simulink model "SimulationModel"  (R2015a)
settings: Solver=ode3  SolverMode=SingleTasking  StartTime=0.0  StopTime=180  FixedStep=Ts  RelTol=1e-3
PostLoadFcn:
  | loadRobotParameters
StartFcn:
  | reset(SimDisplay.getInstance());
undefined symbols (not defined in the file): AxleLength, do_one_run, EncL_init, EncR_init, EncRes, lcam, motorL, motorR, motorX, pcam, SitesPositions, slip_intensity, startPos, TauMotor, theta0, Ts, WheelRadius
libraries: pil_lib x2, simulink x1, realtime_pacer_lib x1, cstblocks x1
CloseFcn:
  | delete(SimDisplay.getInstance());
settings Model: PauseTimes=14  CovSFcnEnable=off  ExtModeTrigDuration=2  Creator=gpacitti  LastModifiedBy=Ye
settings DataIOCC: SaveOutput=off  DSMLogging=off  SaveTime=off
settings OptimizationCC: ExpressionDepthLimit=2147483647  OptimizeModelRefInitCode=on  LifeSpan=1  MaxStackSize=64
settings DebuggingCC: UnderspecifiedInitializationDetection=Classic  MergeDetectMultiDrivingBlocksExec=none  MultiTaskDSMMsg=warning  MultiTaskCondExecSysMsg=none  ParameterPrecisionLossMsg=none  StateNameClashWarn=warning
settings HardwareCC: ProdLargestAtomicInteger=Long  ProdLargestAtomicFloat=Double  ProdEndianess=LittleEndian  ProdHWDeviceType=ARM Compatible->ARM Cortex
settings RTWCC: SystemTargetFile=ert.tlc  TLCOptions=-aInlineSetEventsForThisBaseRateFcn=TLC_FALSE -aSuppressMultiTaskScheduler=TLC_FALSE  TemplateMakefile=ert_default_tmf  Description=Embedded Coder  RTWVerbose=off  Toolchain=GNU Tools for ARM Embedded Processors  CreateSILPILBlock=PIL  CodeExecutionProfiling=on  CodeProfilingSaveOptions=AllData
settings CodeAppCC: IgnoreCustomStorageClasses=off  CustomSymbolStrType=$N$R$M  InternalIdentifier=Classic
settings ERTTargetCC: CodeReplacementLibrary=ARM Cortex-M  GenerateSampleERTMain=off  ParMdlRefBuildCompliant=on  CompOptLevelCompliant=on  ConcurrentExecutionCompliant=on  ERTFirstTimeCompliant=on  SupportContinuousTime=off  ModelStepFunctionPrototypeControlCompliant=on  CPPClassGenCompliant=on  InlinedParameterPlacement=Hierarchical
settings ConfigComp: Description=Design Verifier Custom Configuration Component  DVMaxTestCaseSteps=500  DVTestSuiteOptimization=CombinedObjectives (Nonlinear Extended)  DVDetectActiveLogic=on

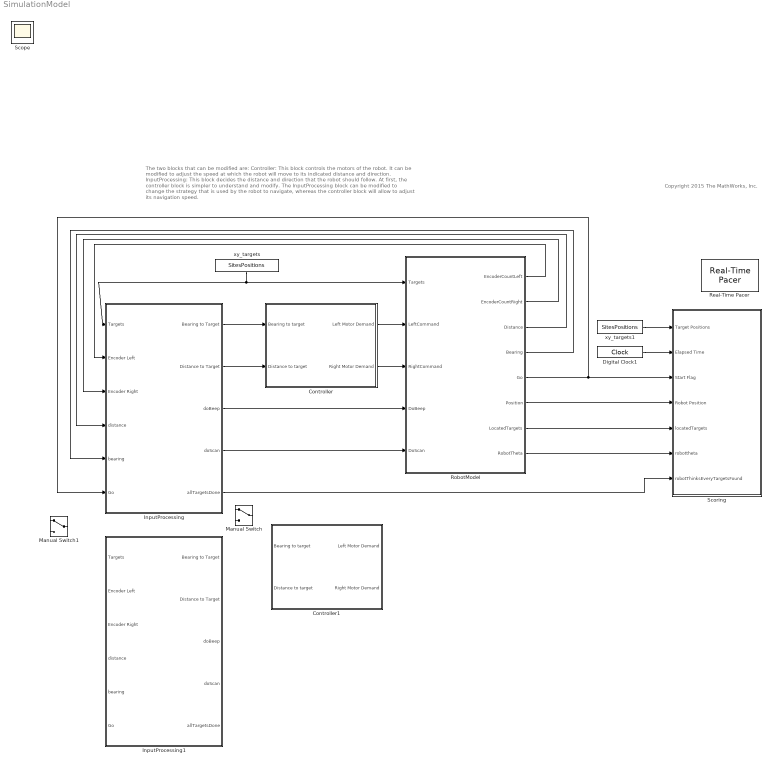
== system SimulationModel ==
  note: Copyright 2015 The MathWorks, Inc.
  note: The two blocks that can be modified are:
      | Controller: This block controls the motors of the robot. It can be modified to adjust the speed at which the robot will move to its indicated distance and direction.
      | InputProcessing: This block decides the distance and direction that the robot should follow.
      |
      | At first, the controller block is simpler to understand and modify.
      | The InputProcessing block can be modified to change the strategy that is used by the robot to navigate, whereas the controller block will allow to adjust its navigation speed.
  Controller : Subsystem  TreatAsAtomicUnit=on
      mask Display: image('Arduino_Mega_2560.jpg',[0.75/2,0.3,0.25,0.4]);
  Controller1 : Subsystem  DialogController=pil_create_dialog  LoadFcn=|
      | try
      |    if ~strcmp(rtw.pil.getPILVersion, '6.8 (R2015a)_12')
      |       set_param(gcb, 'DialogController', '');
      |       set_param(gcb, 'DialogControllerArgs', '');
      |    end
      | catch e
      |       set_param(gcb, 'DialogController', '');
      |       set_param(gcb, 'DialogControllerArgs', '');
      | end
      mask help: PIL:pil:XILBlockMaskDesc
      mask Display: disp('PIL');
  Digital Clock1 : DigitalClock  SampleTime=Ts
  InputProcessing : Subsystem
      mask Display: image('Arduino_Mega_2560.jpg',[0.75/2,0.3,0.25,0.3]);
  InputProcessing1 : Subsystem  DialogController=pil_create_dialog  LoadFcn=|
      | try
      |    if ~strcmp(rtw.pil.getPILVersion, '6.8 (R2015a)_12')
      |       set_param(gcb, 'DialogController', '');
      |       set_param(gcb, 'DialogControllerArgs', '');
      |    end
      | catch e
      |       set_param(gcb, 'DialogController', '');
      |       set_param(gcb, 'DialogControllerArgs', '');
      | end
      mask help: PIL:pil:XILBlockMaskDesc
      mask Display: disp('PIL');
  Manual Switch : ManualSwitch
  Manual Switch1 : ManualSwitch
  Real-Time Pacer : realtime_pacer_lib/Real-Time Pacer  simTimePerRealTime=1
  RobotModel : Subsystem
      mask Display: image('robot_3d.jpg',[0.25,0.35,0.45,0.25]);
  Scoring : Subsystem
      mask Display: image('juge.jpg',[0.45,0.3,0.5,0.25]);
  xy_targets : Constant  Value=SitesPositions  OutDataTypeStr=single
  xy_targets1 : Constant  Value=SitesPositions  OutDataTypeStr=single
  Scope : Scope
      settings: MaxDataPoints=7500
  wires:
  RobotModel/2(EncoderCountRight) -> InputProcessing/3(Encoder Right)
  RobotModel/1(EncoderCountLeft) -> InputProcessing/2(Encoder Left)
  xy_targets/1 -> InputProcessing/1(Targets), RobotModel/1(Targets)
  RobotModel/6(Position) -> Scoring/4(Robot Position)
  InputProcessing/2(Distance to Target) -> Controller/2(Distance to target)
  InputProcessing/1(Bearing to Target) -> Controller/1(Bearing to target)
  Controller/1(Left Motor Demand) -> RobotModel/2(LeftCommand)
  Controller/2(Right Motor Demand) -> RobotModel/3(RightCommand)
  RobotModel/5(Go) -> InputProcessing/6(Go), Scoring/3(Start Flag)
  Digital Clock1/1 -> Scoring/2(Elapsed Time)
  RobotModel/3(Distance) -> InputProcessing/4(distance)
  RobotModel/4(Bearing) -> InputProcessing/5(bearing)
  RobotModel/7(LocatedTargets) -> Scoring/5(locatedTargets)
  RobotModel/8(RobotTheta) -> Scoring/6(robottheta)
  InputProcessing/5(allTargetsDone) -> Scoring/7(robotThinksEveryTargetsFound)
  xy_targets1/1 -> Scoring/1(Target Positions)
  InputProcessing/3(doBeep) -> RobotModel/4(DoBeep)
  InputProcessing/4(doScan) -> RobotModel/5(DoScan)

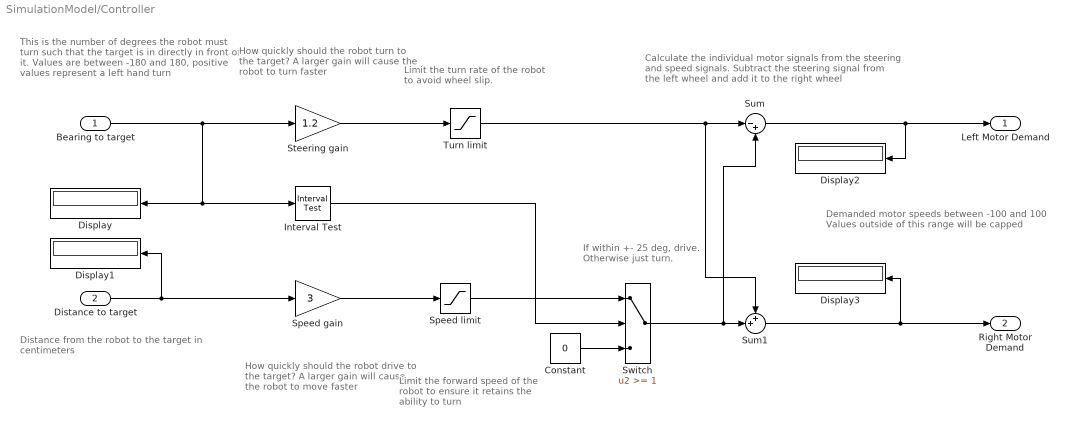
== system SimulationModel/Controller ==
  note: This is the number of degrees the robot
      | must turn such that the target is in directly
      | in front of it.
      | Values are between -180 and 180,
      | positive values represent a left hand turn
  note: Distance from the robot to the target
      | in centimeters
  note: Demanded motor speeds between -100 and 100
      | Values outside of this range will be capped
  note: How quickly should the robot turn
      | to the target? A larger gain will
      |  cause the robot to turn faster
  note: How quickly should the robot
      | drive to the target? A larger gain
      | will cause the robot to move
      | faster
  note: Limit the forward speed of the
      | robot to ensure it retains the
      | ability to turn
  note: Calculate the individual motor signals from the
      | steering and speed signals. Subtract the steering
      | signal from the left wheel and add it to the right
      | wheel
  note: If within +- 25 deg, drive.
      | Otherwise just turn.
  note: Limit the turn rate of the
      | robot to avoid wheel slip.
  Bearing to target : Inport  OutDataTypeStr=single
  Distance to target : Inport  Port=2  PortDimensions=1  SampleTime=Ts
  Constant : Constant  Value=0  OutDataTypeStr=single
  Display{,1..3} (4 alike) : Display
  Interval Test : simulink/Logic and Bit Operations/Interval Test  IntervalClosedRight=on  uplimit=25  IntervalClosedLeft=on  lowlimit=-25  OutDataTypeStr=boolean
      settings: AttributesFormatString=|
      | Upper = %<uplimit>
      | Lower = %<lowlimit>
  Speed gain : Gain  Gain=3
  Speed limit : Saturate  UpperLimit=40  LowerLimit=0
      settings: AttributesFormatString=|
      | Upper = %<UpperLimit>
      | Lower = %<LowerLimit>
  Steering gain : Gain  Gain=1.2
  Sum : Sum  Inputs=|-+
  Sum1 : Sum  Inputs=++|
  Switch : Switch  Threshold=1
  Turn limit : Saturate  UpperLimit=50  LowerLimit=-50
      settings: AttributesFormatString=|
      | Upper = %<UpperLimit>
      | Lower = %<LowerLimit>
  Left Motor Demand : Outport  OutDataTypeStr=single
  Right Motor Demand : Outport  Port=2  OutDataTypeStr=single
  wires:
  Speed limit/1 -> Switch/1
  Turn limit/1 -> Sum1/1, Sum/1
  Constant/1 -> Switch/3
  Interval Test/1 -> Switch/2
  Switch/1 -> Sum1/2, Sum/2
  Sum/1 -> Display2/1, Left Motor Demand/1
  Sum1/1 -> Display3/1, Right Motor Demand/1
  Steering gain/1 -> Turn limit/1
  Distance to target/1 -> Speed gain/1, Display1/1
  Speed gain/1 -> Speed limit/1
  Bearing to target/1 -> Interval Test/1, Display/1, Steering gain/1

== system SimulationModel/Controller1 ==
  Bearing to target : Inport  OutDataTypeStr=single
  Distance to target : Inport  Port=2  PortDimensions=1  SampleTime=Ts
  Controller_sfcn : pil_lib/PIL Block  SimulationMode=PIL  IsTopModelPIL=off  CodeDir=D:\Dropbox\Phd\AutomaticScriptForSubRegions\MarsRover2014\work\Controller_ert_rtw  ConfigName=ARM Cortex-M3 (QEMU)
  __InputSSForSFun__ : Subsystem
  __OutputSSForSFun__ : Subsystem
  Left Motor Demand : Outport  OutDataTypeStr=single
  Right Motor Demand : Outport  Port=2  OutDataTypeStr=single
  wires:
  __OutputSSForSFun__/2(Right Motor Demand) -> Right Motor Demand/1
  __OutputSSForSFun__/1(Left Motor Demand) -> Left Motor Demand/1
  Controller_sfcn/2 -> __OutputSSForSFun__/2(__UniqueInportName__2__)
  Controller_sfcn/1 -> __OutputSSForSFun__/1(__UniqueInportName__1__)
  __InputSSForSFun__/2(__UniqueOutportName__2__) -> Controller_sfcn/2
  __InputSSForSFun__/1(__UniqueOutportName__1__) -> Controller_sfcn/1
  Distance to target/1 -> __InputSSForSFun__/2(Distance to target)
  Bearing to target/1 -> __InputSSForSFun__/1(Bearing to target)

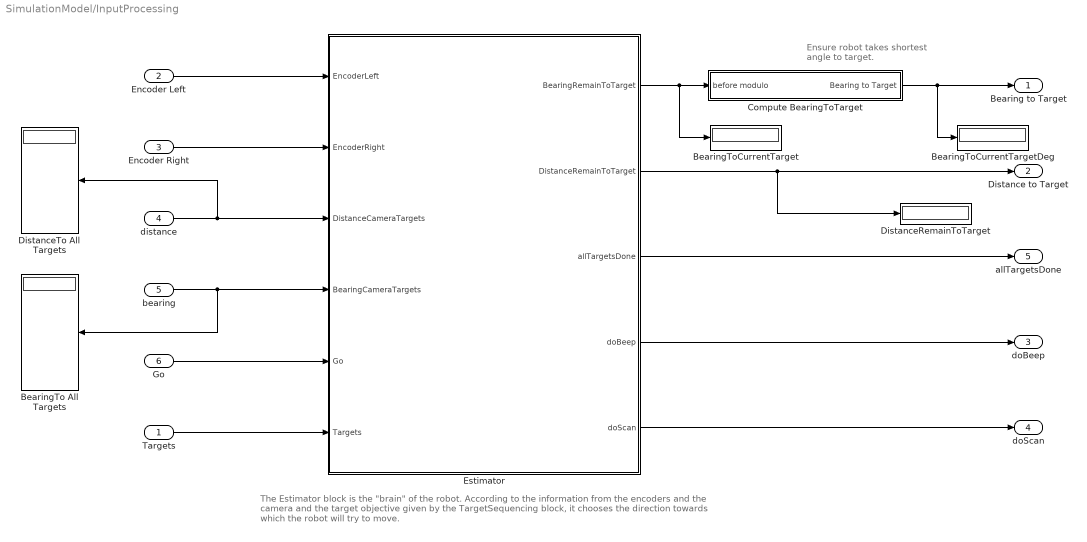
== system SimulationModel/InputProcessing ==
  note: The Estimator block is the "brain" of the robot. According to the information from the encoders and the camera and the
      | target objective given by the TargetSequencing block, it chooses the direction towards which the robot will try to move.
  note: Ensure robot takes shortest
      | angle to target.
  Targets : Inport
  Encoder Left : Inport  Port=2  OutDataTypeStr=int32
  Encoder Right : Inport  Port=3  OutDataTypeStr=int32
  distance : Inport  Port=4
  bearing : Inport  Port=5
  Go : Inport  Port=6
  BearingTo All Targets : Display
  BearingToCurrentTarget : Display
  BearingToCurrentTargetDeg : Display
  Compute BearingToTarget : Subsystem
  DistanceRemainToTarget : Display
  DistanceTo All Targets : Display
  Estimator : Stateflow chart  TreatAsAtomicUnit=on
  Bearing to Target : Outport  SampleTime=Ts
  Distance to Target : Outport  Port=2
  doBeep : Outport  Port=3
  doScan : Outport  Port=4
  allTargetsDone : Outport  Port=5
  wires:
  distance/1 -> DistanceTo All Targets/1, Estimator/3(DistanceCameraTargets)
  bearing/1 -> BearingTo All Targets/1, Estimator/4(BearingCameraTargets)
  Compute BearingToTarget/1(Bearing to Target) -> BearingToCurrentTargetDeg/1, Bearing to Target/1
  Estimator/2(DistanceRemainToTarget) -> DistanceRemainToTarget/1, Distance to Target/1
  Estimator/1(BearingRemainToTarget) -> Compute BearingToTarget/1(before modulo), BearingToCurrentTarget/1
  Encoder Right/1 -> Estimator/2(EncoderRight)
  Encoder Left/1 -> Estimator/1(EncoderLeft)
  Targets/1 -> Estimator/6(Targets)
  Go/1 -> Estimator/5(Go)
  Estimator/3(allTargetsDone) -> allTargetsDone/1
  Estimator/4(doBeep) -> doBeep/1
  Estimator/5(doScan) -> doScan/1

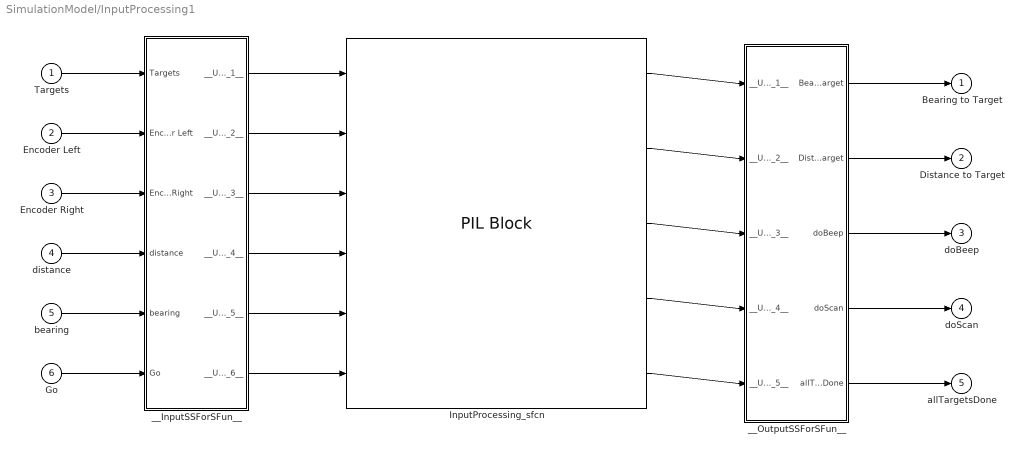
== system SimulationModel/InputProcessing1 ==
  Targets : Inport
  Encoder Left : Inport  Port=2  OutDataTypeStr=int32
  Encoder Right : Inport  Port=3  OutDataTypeStr=int32
  distance : Inport  Port=4
  bearing : Inport  Port=5
  Go : Inport  Port=6
  InputProcessing_sfcn : pil_lib/PIL Block  SimulationMode=PIL  IsTopModelPIL=off  CodeDir=D:\Dropbox\Phd\AutomaticScriptForSubRegions\MarsRover2014\work\InputProcessing_ert_rtw  ConfigName=ARM Cortex-M3 (QEMU)
  __InputSSForSFun__ : Subsystem
  __OutputSSForSFun__ : Subsystem
  Bearing to Target : Outport  SampleTime=Ts
  Distance to Target : Outport  Port=2
  doBeep : Outport  Port=3
  doScan : Outport  Port=4
  allTargetsDone : Outport  Port=5
  wires:
  __OutputSSForSFun__/5(allTargetsDone) -> allTargetsDone/1
  __OutputSSForSFun__/4(doScan) -> doScan/1
  __OutputSSForSFun__/3(doBeep) -> doBeep/1
  __OutputSSForSFun__/2(Distance to Target) -> Distance to Target/1
  __OutputSSForSFun__/1(Bearing to Target) -> Bearing to Target/1
  InputProcessing_sfcn/5 -> __OutputSSForSFun__/5(__UniqueInportName__5__)
  InputProcessing_sfcn/4 -> __OutputSSForSFun__/4(__UniqueInportName__4__)
  InputProcessing_sfcn/3 -> __OutputSSForSFun__/3(__UniqueInportName__3__)
  InputProcessing_sfcn/2 -> __OutputSSForSFun__/2(__UniqueInportName__2__)
  InputProcessing_sfcn/1 -> __OutputSSForSFun__/1(__UniqueInportName__1__)
  __InputSSForSFun__/6(__UniqueOutportName__6__) -> InputProcessing_sfcn/6
  __InputSSForSFun__/5(__UniqueOutportName__5__) -> InputProcessing_sfcn/5
  __InputSSForSFun__/4(__UniqueOutportName__4__) -> InputProcessing_sfcn/4
  __InputSSForSFun__/3(__UniqueOutportName__3__) -> InputProcessing_sfcn/3
  __InputSSForSFun__/2(__UniqueOutportName__2__) -> InputProcessing_sfcn/2
  __InputSSForSFun__/1(__UniqueOutportName__1__) -> InputProcessing_sfcn/1
  Go/1 -> __InputSSForSFun__/6(Go)
  bearing/1 -> __InputSSForSFun__/5(bearing)
  distance/1 -> __InputSSForSFun__/4(distance)
  Encoder Right/1 -> __InputSSForSFun__/3(Encoder Right)
  Encoder Left/1 -> __InputSSForSFun__/2(Encoder Left)
  Targets/1 -> __InputSSForSFun__/1(Targets)

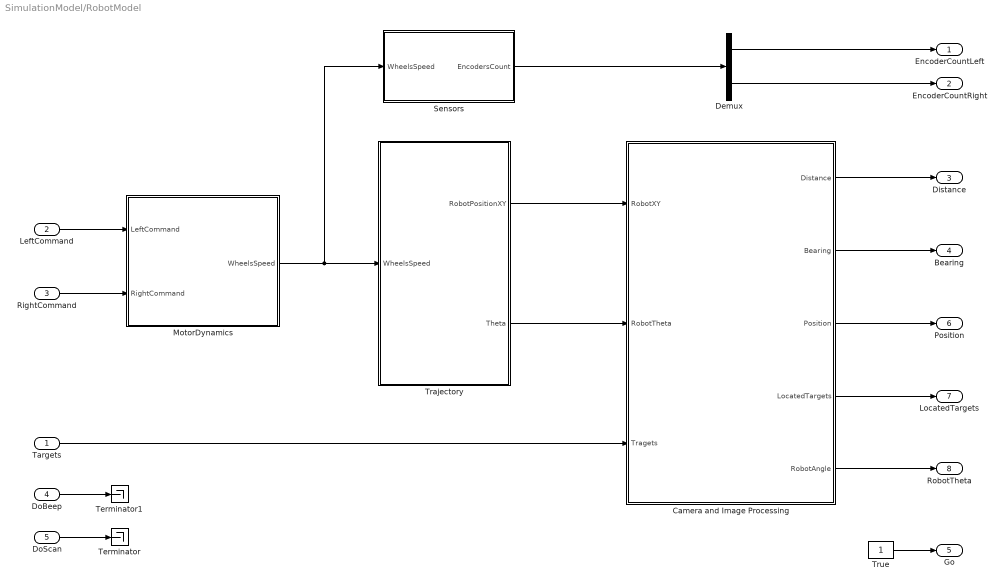
== system SimulationModel/RobotModel ==
  Targets : Inport
  LeftCommand : Inport  Port=2  SampleTime=0
  RightCommand : Inport  Port=3  SampleTime=0
  DoBeep : Inport  Port=4  SampleTime=0
  DoScan : Inport  Port=5  SampleTime=0
  Camera and Image Processing : Subsystem
  Demux : Demux  Outputs=2
  MotorDynamics : Subsystem
  Sensors : Subsystem
  Terminator : Terminator
  Terminator1 : Terminator
  Trajectory : Subsystem
  True : Constant  OutMin=0  OutMax=1  OutDataTypeStr=boolean  SampleTime=0.1
  EncoderCountLeft : Outport  OutDataTypeStr=int32
  EncoderCountRight : Outport  Port=2  OutDataTypeStr=int32
  Distance : Outport  Port=3  OutDataTypeStr=int16
  Bearing : Outport  Port=4  OutDataTypeStr=int8
  Go : Outport  Port=5
  Position : Outport  Port=6
  LocatedTargets : Outport  Port=7
  RobotTheta : Outport  Port=8
  wires:
  Trajectory/2(Theta) -> Camera and Image Processing/2(RobotTheta)
  True/1 -> Go/1
  DoScan/1 -> Terminator/1
  DoBeep/1 -> Terminator1/1
  MotorDynamics/1(WheelsSpeed) -> Trajectory/1(WheelsSpeed), Sensors/1(WheelsSpeed)
  LeftCommand/1 -> MotorDynamics/1(LeftCommand)
  RightCommand/1 -> MotorDynamics/2(RightCommand)
  Sensors/1(EncodersCount) -> Demux/1
  Demux/1 -> EncoderCountLeft/1
  Demux/2 -> EncoderCountRight/1
  Targets/1 -> Camera and Image Processing/3(Tragets)
  Camera and Image Processing/1(Distance) -> Distance/1
  Camera and Image Processing/2(Bearing) -> Bearing/1
  Camera and Image Processing/3(Position) -> Position/1
  Camera and Image Processing/4(LocatedTargets) -> LocatedTargets/1
  Camera and Image Processing/5(RobotAngle) -> RobotTheta/1
  Trajectory/1(RobotPositionXY) -> Camera and Image Processing/1(RobotXY)

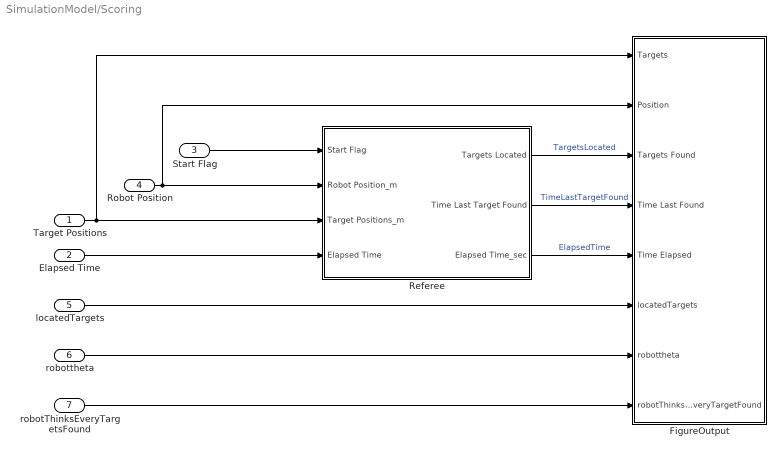
== system SimulationModel/Scoring ==
  Target Positions : Inport
  Elapsed Time : Inport  Port=2
  Start Flag : Inport  Port=3
  Robot Position : Inport  Port=4
  locatedTargets : Inport  Port=5
  robottheta : Inport  Port=6
  robotThinksEveryTargetsFound : Inport  Port=7
  FigureOutput : Subsystem  TreatAsAtomicUnit=on  SimViewingDevice=on
  Referee : Subsystem
      mask Display: % image(imread('referee.png'))
  wires:
  Referee/1(Targets Located) -> FigureOutput/3(Targets Found)  "TargetsLocated"
  Referee/2(Time Last Target Found) -> FigureOutput/4(Time Last Found)  "TimeLastTargetFound"
  Referee/3(Elapsed Time_sec) -> FigureOutput/5(Time Elapsed)  "ElapsedTime"
  Start Flag/1 -> Referee/1(Start Flag)
  Robot Position/1 -> Referee/2(Robot Position_m), FigureOutput/2(Position)
  Elapsed Time/1 -> Referee/4(Elapsed Time)
  Target Positions/1 -> FigureOutput/1(Targets), Referee/3(Target Positions_m)
  locatedTargets/1 -> FigureOutput/6(locatedTargets)
  robottheta/1 -> FigureOutput/7(robottheta)
  robotThinksEveryTargetsFound/1 -> FigureOutput/8(robotThinksEveryTargetFound)

== system SimulationModel/Controller1/__InputSSForSFun__ ==
  Bearing to target : Inport  OutDataTypeStr=single
  Distance to target : Inport  Port=2  PortDimensions=1  SampleTime=Ts
  __UniqueOutportName__1__ : Outport
  __UniqueOutportName__2__ : Outport  Port=2
  wires:
  Distance to target/1 -> __UniqueOutportName__2__/1
  Bearing to target/1 -> __UniqueOutportName__1__/1

== system SimulationModel/Controller1/__OutputSSForSFun__ ==
  __UniqueInportName__1__ : Inport
  __UniqueInportName__2__ : Inport  Port=2
  Left Motor Demand : Outport  OutDataTypeStr=single
  Right Motor Demand : Outport  Port=2  OutDataTypeStr=single
  wires:
  __UniqueInportName__2__/1 -> Right Motor Demand/1
  __UniqueInportName__1__/1 -> Left Motor Demand/1

== system SimulationModel/InputProcessing/Compute BearingToTarget ==
  before modulo : Inport
  Constant : Constant  Value=180  OutDataTypeStr=Inherit: Inherit via back propagation
  Constant1 : Constant  Value=360  OutDataTypeStr=Inherit: Inherit via back propagation
  Math Function1 : Math  Operator=mod  SaturateOnIntegerOverflow=on
  Sum10 : Sum  Inputs=-+|
  Sum7 : Sum  Inputs=++|
  Bearing to Target : Outport  SampleTime=Ts
  wires:
  before modulo/1 -> Sum7/2
  Sum10/1 -> Bearing to Target/1
  Math Function1/1 -> Sum10/2
  Constant1/1 -> Math Function1/2
  Sum7/1 -> Math Function1/1
  Constant/1 -> Sum10/1, Sum7/1

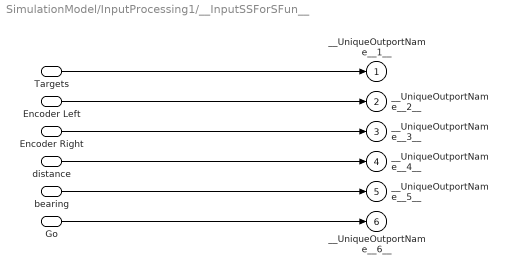
== system SimulationModel/InputProcessing1/__InputSSForSFun__ ==
  Targets : Inport
  Encoder Left : Inport  Port=2  OutDataTypeStr=int32
  Encoder Right : Inport  Port=3  OutDataTypeStr=int32
  distance : Inport  Port=4
  bearing : Inport  Port=5
  Go : Inport  Port=6
  __UniqueOutportName__1__ : Outport
  __UniqueOutportName__2__ : Outport  Port=2
  __UniqueOutportName__3__ : Outport  Port=3
  __UniqueOutportName__4__ : Outport  Port=4
  __UniqueOutportName__5__ : Outport  Port=5
  __UniqueOutportName__6__ : Outport  Port=6
  wires:
  Go/1 -> __UniqueOutportName__6__/1
  bearing/1 -> __UniqueOutportName__5__/1
  distance/1 -> __UniqueOutportName__4__/1
  Encoder Right/1 -> __UniqueOutportName__3__/1
  Encoder Left/1 -> __UniqueOutportName__2__/1
  Targets/1 -> __UniqueOutportName__1__/1

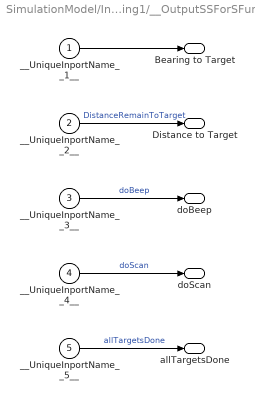
== system SimulationModel/InputProcessing1/__OutputSSForSFun__ ==
  __UniqueInportName__1__ : Inport
  __UniqueInportName__2__ : Inport  Port=2
  __UniqueInportName__3__ : Inport  Port=3
  __UniqueInportName__4__ : Inport  Port=4
  __UniqueInportName__5__ : Inport  Port=5
  Bearing to Target : Outport  SampleTime=Ts
  Distance to Target : Outport  Port=2
  doBeep : Outport  Port=3
  doScan : Outport  Port=4
  allTargetsDone : Outport  Port=5
  wires:
  __UniqueInportName__5__/1 -> allTargetsDone/1  "allTargetsDone"
  __UniqueInportName__4__/1 -> doScan/1  "doScan"
  __UniqueInportName__3__/1 -> doBeep/1  "doBeep"
  __UniqueInportName__2__/1 -> Distance to Target/1  "DistanceRemainToTarget"
  __UniqueInportName__1__/1 -> Bearing to Target/1

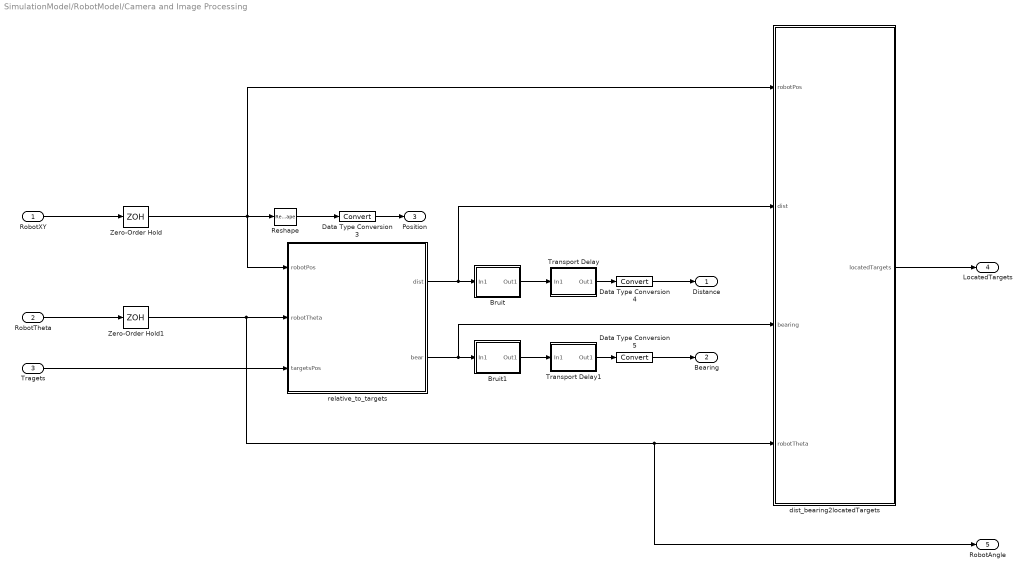
== system SimulationModel/RobotModel/Camera and Image Processing ==
  RobotXY : Inport
  RobotTheta : Inport  Port=2
  Tragets : Inport  Port=3
  Bruit : Subsystem
  Bruit1 : Subsystem
  Data Type Conversion3 : DataTypeConversion
  Data Type Conversion4 : DataTypeConversion
  Data Type Conversion5 : DataTypeConversion
  Reshape : Reshape  OutputDimensionality=Row vector (2-D)
  Transport Delay : Subsystem  mask{timeDelay=0.300, initialOutput=zeros(size(6,1),1), initialBufferSize=1024, useFixedBufferSize=off, directFeedthoughOfInputDuringLinearization=off, padeOrder=0}
      mask prompts: initialOutput "Initial output"; initialBufferSize "Initial buffer size"; useFixedBufferSize "Use fixed buffer size"; directFeedthoughOfInputDuringLinearization "Direct feedthough of input during linearization"; padeOrder "Pade order (for linearization):"
  Transport Delay1 : Subsystem  mask{timeDelay=0.300, initialOutput=zeros(size(6,1),1), initialBufferSize=1024, useFixedBufferSize=off, directFeedthoughOfInputDuringLinearization=off, padeOrder=0}
      mask prompts: initialOutput "Initial output"; initialBufferSize "Initial buffer size"; useFixedBufferSize "Use fixed buffer size"; directFeedthoughOfInputDuringLinearization "Direct feedthough of input during linearization"; padeOrder "Pade order (for linearization):"
  Zero-Order Hold : ZeroOrderHold  SampleTime=Ts
  Zero-Order Hold1 : ZeroOrderHold  SampleTime=Ts
  dist_bearing2locatedTargets : MATLAB Function  TreatAsAtomicUnit=on
  relative_to_targets : MATLAB Function  TreatAsAtomicUnit=on
  Distance : Outport  OutDataTypeStr=int16
  Bearing : Outport  Port=2  OutDataTypeStr=int8
  Position : Outport  Port=3
  LocatedTargets : Outport  Port=4
  RobotAngle : Outport  Port=5
  wires:
  RobotTheta/1 -> Zero-Order Hold1/1
  RobotXY/1 -> Zero-Order Hold/1
  Bruit/1(Out1) -> Transport Delay/1(In1)
  Transport Delay1/1(Out1) -> Data Type Conversion5/1
  Tragets/1 -> relative_to_targets/3(targetsPos)
  Data Type Conversion4/1 -> Distance/1
  Transport Delay/1(Out1) -> Data Type Conversion4/1
  Data Type Conversion5/1 -> Bearing/1
  Data Type Conversion3/1 -> Position/1
  Bruit1/1(Out1) -> Transport Delay1/1(In1)
  relative_to_targets/1(dist) -> dist_bearing2locatedTargets/2(dist), Bruit/1(In1)
  Reshape/1 -> Data Type Conversion3/1
  relative_to_targets/2(bear) -> dist_bearing2locatedTargets/3(bearing), Bruit1/1(In1)
  dist_bearing2locatedTargets/1(locatedTargets) -> LocatedTargets/1
  Zero-Order Hold/1 -> relative_to_targets/1(robotPos), dist_bearing2locatedTargets/1(robotPos), Reshape/1
  Zero-Order Hold1/1 -> RobotAngle/1, dist_bearing2locatedTargets/4(robotTheta), relative_to_targets/2(robotTheta)

== system SimulationModel/RobotModel/MotorDynamics ==
  LeftCommand : Inport
  RightCommand : Inport  Port=2
  Dynamics : cstblocks/LTI System  sys=tf(1,[TauMotor 1])*eye(2)  IC=[]
  Left_motor_table : Lookup_n-D  NumberOfTableDimensions=1  BreakpointsForDimension1=motorX  Table=motorL  ExtrapMethod=Clip  InternalRulePriority=Speed  OutDataTypeStr=Inherit: Inherit via back propagation  RndMeth=Simplest  InputSameDT=on
  Mux1 : Mux  Inputs=2
  Right_motor_table : Lookup_n-D  NumberOfTableDimensions=1  BreakpointsForDimension1=motorX  Table=motorR  ExtrapMethod=Clip  InternalRulePriority=Speed  OutDataTypeStr=Inherit: Inherit via back propagation  RndMeth=Simplest  InputSameDT=on
  WheelsSpeed : Outport  PortDimensions=2
  wires:
  Dynamics/1 -> WheelsSpeed/1  "Wheels Velocity d°/s"
  LeftCommand/1 -> Left_motor_table/1
  RightCommand/1 -> Right_motor_table/1
  Right_motor_table/1 -> Mux1/2
  Left_motor_table/1 -> Mux1/1
  Mux1/1 -> Dynamics/1  "Speed Demand d°/s"

== system SimulationModel/RobotModel/Sensors ==
  WheelsSpeed : Inport
  Data Type Conversion : DataTypeConversion
  Encoder Quantization : Quantizer  QuantizationInterval=(360/EncRes)
  Encoder Reading : ZeroOrderHold  SampleTime=Ts
  Integrator : Integrator  InitialCondition=[EncL_init;EncR_init]
  deg2encoderCount : Gain  Gain=EncRes/360  OutDataTypeStr=Inherit: Inherit via back propagation
  EncodersCount : Outport
  wires:
  deg2encoderCount/1 -> Data Type Conversion/1
  WheelsSpeed/1 -> Integrator/1  "Wheels Velocity d°/s"
  Encoder Quantization/1 -> deg2encoderCount/1
  Data Type Conversion/1 -> EncodersCount/1
  Encoder Reading/1 -> Encoder Quantization/1
  Integrator/1 -> Encoder Reading/1  "WheelsPosition d°"

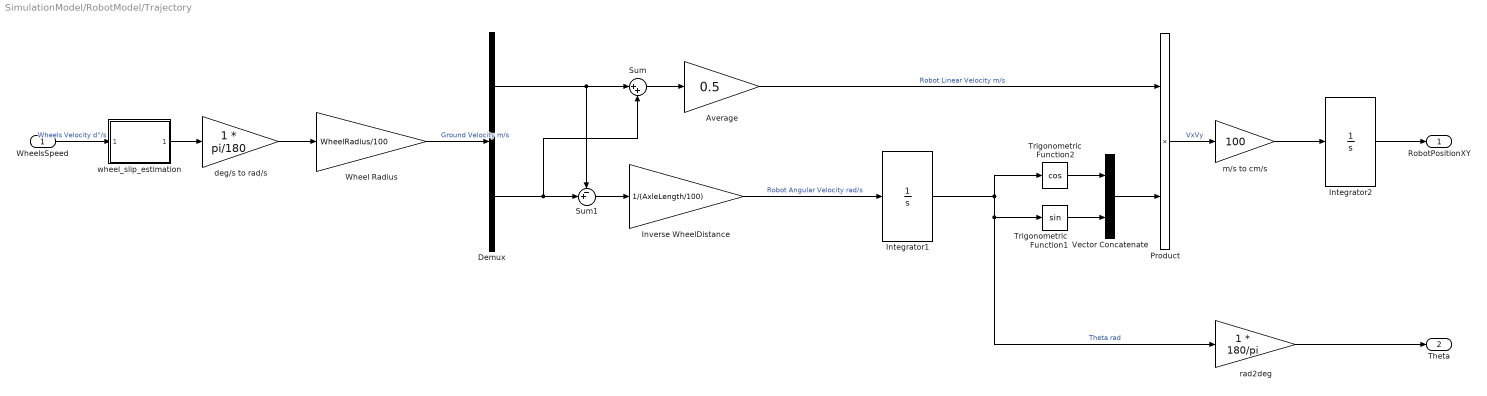
== system SimulationModel/RobotModel/Trajectory ==
  WheelsSpeed : Inport  PortDimensions=2
  Average : Gain  Gain=0.5
  Demux : Demux  Outputs=2
  Integrator1 : Integrator  InitialCondition=theta0 * pi/180
  Integrator2 : Integrator  InitialCondition=startPos
  Inverse WheelDistance : Gain  Gain=1/(AxleLength/100)
  Product : Product
  Sum : Sum  Inputs=|++
  Sum1 : Sum  Inputs=-+|
  Trigonometric Function1 : Trigonometry
  Trigonometric Function2 : Trigonometry  Operator=cos
  Vector Concatenate : Concatenate
  Wheel Radius : Gain  Gain=WheelRadius/100
  deg/s to rad/s : Gain  Gain=1 * pi/180
  m/s to cm/s : Gain  Gain=100
  rad2deg : Gain  Gain=1 * 180/pi
  wheel_slip_estimation : Subsystem  mask(Wheel slip){slip_intensity=slip_intensity}
      mask prompts: slip_intensity "Slip intensity"
      mask help: Add slip in wheel speed
  RobotPositionXY : Outport
  Theta : Outport  Port=2
  wires:
  Integrator1/1 -> rad2deg/1, Trigonometric Function1/1, Trigonometric Function2/1  "Theta rad"
  Trigonometric Function2/1 -> Vector Concatenate/1
  Trigonometric Function1/1 -> Vector Concatenate/2
  Vector Concatenate/1 -> Product/2
  Wheel Radius/1 -> Demux/1  "Ground Velocity m/s"
  Average/1 -> Product/1  "Robot Linear Velocity m/s"
  Sum/1 -> Average/1
  Demux/2 -> Sum1/2, Sum/2
  Demux/1 -> Sum1/1, Sum/1
  Sum1/1 -> Inverse WheelDistance/1
  Product/1 -> m/s to cm/s/1  "VxVy"
  Inverse WheelDistance/1 -> Integrator1/1  "Robot Angular Velocity rad/s"
  deg/s to rad/s/1 -> Wheel Radius/1
  m/s to cm/s/1 -> Integrator2/1
  Integrator2/1 -> RobotPositionXY/1
  rad2deg/1 -> Theta/1
  WheelsSpeed/1 -> wheel_slip_estimation/1(perfect_wheel_velocity_degps)  "Wheels Velocity d°/s"
  wheel_slip_estimation/1(real_wheel_velocity_degps) -> deg/s to rad/s/1

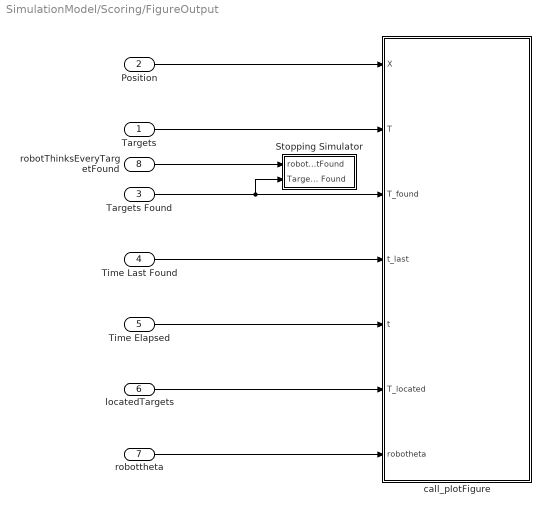
== system SimulationModel/Scoring/FigureOutput ==
  Targets : Inport
  Position : Inport  Port=2
  Targets Found : Inport  Port=3
  Time Last Found : Inport  Port=4
  Time Elapsed : Inport  Port=5
  locatedTargets : Inport  Port=6
  robottheta : Inport  Port=7
  robotThinksEveryTargetFound : Inport  Port=8
  Stopping Simulator : Subsystem
  call_plotFigure : MATLAB Function  TreatAsAtomicUnit=on
  wires:
  Position/1 -> call_plotFigure/1(X)
  Targets/1 -> call_plotFigure/2(T)
  Targets Found/1 -> call_plotFigure/3(T_found), Stopping Simulator/2(Targets Found)
  Time Last Found/1 -> call_plotFigure/4(t_last)
  Time Elapsed/1 -> call_plotFigure/5(t)
  locatedTargets/1 -> call_plotFigure/6(T_located)
  robottheta/1 -> call_plotFigure/7(robotheta)
  robotThinksEveryTargetFound/1 -> Stopping Simulator/1(robotThinksEveryTargetFound)

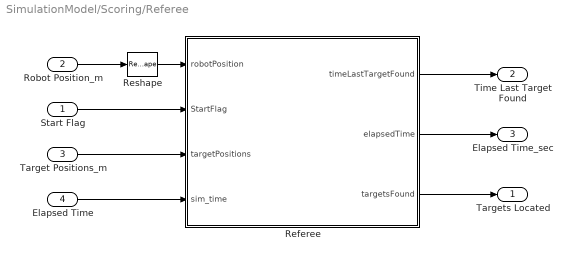
== system SimulationModel/Scoring/Referee ==
  Start Flag : Inport  OutDataTypeStr=boolean  SampleTime=Ts
  Robot Position_m : Inport  Port=2  SampleTime=Ts
  Target Positions_m : Inport  Port=3  SampleTime=Ts
  Elapsed Time : Inport  Port=4  SampleTime=Ts
  Referee : Stateflow chart  TreatAsAtomicUnit=on
  Reshape : Reshape  OutputDimensionality=Row vector (2-D)
  Targets Located : Outport
  Time Last Target Found : Outport  Port=2  PortDimensions=1
  Elapsed Time_sec : Outport  Port=3  PortDimensions=1
  wires:
  Referee/1(timeLastTargetFound) -> Time Last Target Found/1
  Referee/3(targetsFound) -> Targets Located/1
  Robot Position_m/1 -> Reshape/1
  Start Flag/1 -> Referee/2(StartFlag)
  Reshape/1 -> Referee/1(robotPosition)
  Target Positions_m/1 -> Referee/3(targetPositions)
  Referee/2(elapsedTime) -> Elapsed Time_sec/1
  Elapsed Time/1 -> Referee/4(sim_time)

== system SimulationModel/RobotModel/Camera and Image Processing/Bruit ==
  In1 : Inport
  Add : Sum
  Data Type Conversion4 : DataTypeConversion
  Product : Product
  Uniform Random Number : UniformRandomNumber  Minimum=-0.05  Maximum=0.05  SampleTime=Ts
  Out1 : Outport
  wires:
  In1/1 -> Add/2, Product/2
  Product/1 -> Add/1
  Uniform Random Number/1 -> Data Type Conversion4/1
  Data Type Conversion4/1 -> Product/1
  Add/1 -> Out1/1

== system SimulationModel/RobotModel/Camera and Image Processing/Bruit1 ==
  In1 : Inport
  Add : Sum
  Data Type Conversion4 : DataTypeConversion
  Product : Product
  Uniform Random Number : UniformRandomNumber  Minimum=-0.05  Maximum=0.05  SampleTime=Ts
  Out1 : Outport
  wires:
  Data Type Conversion4/1 -> Product/1
  Uniform Random Number/1 -> Data Type Conversion4/1
  Product/1 -> Add/1
  In1/1 -> Add/2, Product/2
  Add/1 -> Out1/1

== system SimulationModel/RobotModel/Camera and Image Processing/Transport Delay ==
  In1 : Inport
  Data Type Conversion : DataTypeConversion  OutDataTypeStr=double
  Data Type Conversion4 : DataTypeConversion  OutDataTypeStr=single
  Transport Delay : TransportDelay  DelayTime=timeDelay  InitialOutput=initialOutput  BufferSize=initialBufferSize  PadeOrder=padeOrder
  Zero-Order Hold : ZeroOrderHold  SampleTime=Ts
  Out1 : Outport
  wires:
  Transport Delay/1 -> Data Type Conversion4/1
  Data Type Conversion/1 -> Transport Delay/1
  Data Type Conversion4/1 -> Zero-Order Hold/1
  In1/1 -> Data Type Conversion/1
  Zero-Order Hold/1 -> Out1/1

== system SimulationModel/RobotModel/Camera and Image Processing/Transport Delay1 ==
  In1 : Inport
  Data Type Conversion : DataTypeConversion  OutDataTypeStr=double
  Data Type Conversion4 : DataTypeConversion  OutDataTypeStr=single
  Transport Delay : TransportDelay  DelayTime=timeDelay  InitialOutput=initialOutput  BufferSize=initialBufferSize  PadeOrder=padeOrder
  Zero-Order Hold : ZeroOrderHold  SampleTime=Ts
  Out1 : Outport
  wires:
  In1/1 -> Data Type Conversion/1
  Data Type Conversion4/1 -> Zero-Order Hold/1
  Data Type Conversion/1 -> Transport Delay/1
  Transport Delay/1 -> Data Type Conversion4/1
  Zero-Order Hold/1 -> Out1/1

== system SimulationModel/RobotModel/Trajectory/wheel_slip_estimation ==
  perfect_wheel_velocity_degps : Inport
  Gain : Gain  Gain=1/(pi/4 * slip_intensity)
  Gain1 : Gain  Gain=(pi/4)*slip_intensity
  Trigonometric Function : Trigonometry  Operator=atan
  real_wheel_velocity_degps : Outport
  wires:
  perfect_wheel_velocity_degps/1 -> Gain1/1
  Trigonometric Function/1 -> Gain/1
  Gain1/1 -> Trigonometric Function/1
  Gain/1 -> real_wheel_velocity_degps/1

== system SimulationModel/Scoring/FigureOutput/Stopping Simulator ==
  robotThinksEveryTargetFound : Inport
  Targets Found : Inport  Port=2
  Constant : Constant  Value=do_one_run
  Data Type Conversion : DataTypeConversion  OutDataTypeStr=double
  Logical Operator : Logic  Operator=OR  AllPortsSameDT=off  OutDataTypeStr=boolean
  Logical Operator1 : Logic  AllPortsSameDT=off  OutDataTypeStr=boolean
  MinMax : MinMax
  Stop Simulation : Stop
  wires:
  Targets Found/1 -> Data Type Conversion/1
  Data Type Conversion/1 -> MinMax/1
  robotThinksEveryTargetFound/1 -> Logical Operator/1
  MinMax/1 -> Logical Operator/2
  Logical Operator/1 -> Logical Operator1/1
  Constant/1 -> Logical Operator1/2
  Logical Operator1/1 -> Stop Simulation/1

== stateflow chart SimulationModel/InputProcessing/Estimator ==
  state Standby
    entry:
    %Init
    doBeep = false;doScan = false;
    encoder_left_prev_target = int32(0);
    encoder_right_prev_target = int32(0);
    ind = uint8(0);
    CurrentDistance = single(0);
    prev_target = single(startPos);
    prev_bearing = single(0);
    TargetIndex = uint8(0);
    allTargetsDone = false;
  state Running
    state Next_Target
      entry:
      doScan = false;
      TargetIndex = TargetIndex + 1;
      %Calc relative distance to next target
      DistanceToTarget = norm(Targets(TargetIndex,1:2)-prev_target);
      %Calc relative bearing to next target
      BearingToTarget = atan2d(Targets(TargetIndex,2)-prev_target(2),...
      Targets(TargetIndex,1)-prev_target(1)) - prev_bearing;
      %Save values for relative moves
      prev_target = Targets(TargetIndex,1:2);
      prev_bearing = prev_bearing + BearingToTarget;
      encoder_left_prev_target = EncoderLeft;
      encoder_right_prev_target = EncoderRight;
      DistanceRemainToTarget = DistanceToTarget;
      BearingRemainToTarget = BearingToTarget;
    state Apply_camera_correction
      entry:
      %Find the closest match between seen targets and current destination
      TargetFound = uint8(0);
      dist_remaining = int16(DistanceRemainToTarget);
      for ind=1:uint8(length(DistanceCameraTargets))
      if(DistanceCameraTargets(ind) ~= 0 )
      if(abs(DistanceCameraTargets(ind) - dist_remaining) < 15)
      if (TargetFound == 0 || abs(DistanceCameraTargets(TargetFound) -  ...
      dist_remaining) > abs(DistanceCameraTargets(ind) - dist_remaining))
      TargetFound = uint8(ind);
      end
      end
      end
      end
      %If a target is found update the distance and bearing from the camera
      if ( TargetFound ~= 0 )
      doBeep = true;
      DistanceToTarget = single(DistanceCameraTargets(TargetFound));
      BearingToTarget = single(BearingCameraTargets(TargetFound))/2;
      encoder_left_prev_target = EncoderLeft;
      encoder_right_prev_target = EncoderRight;
      end
    state Wait_for_scoring
      entry:
      DistanceRemainToTarget = single(0);
      doScan = true;
    state Calc_next_robot_move
      entry,during:
      doBeep = false;
      %Calc the new trajectory based on what has already been done
      dL = single(EncoderLeft - encoder_left_prev_target) * 2 * WheelRadius * pi / EncRes;
      dR = single(EncoderRight - encoder_right_prev_target) * 2 * WheelRadius * pi / EncRes;
      CurrentDistance = ((dL + dR)/2);
      CurrentBearing = single(((dR - dL)*180) / (AxleLength*1.01*pi));
      DistanceRemainToTarget = DistanceToTarget - CurrentDistance;
      BearingRemainToTarget = BearingToTarget - CurrentBearing;
    (default) -> Next_Target
    Next_Target -> Calc_next_robot_move
    Wait_for_scoring -> Next_Target : after(3,sec)
    Calc_next_robot_move -> Wait_for_scoring [order 1] : [DistanceRemainToTarget < 7]
    Calc_next_robot_move -> Apply_camera_correction [order 2] : [CurrentDistance > 5 && DistanceRemainToTarget > pcam(1)-5]
    Apply_camera_correction -> Calc_next_robot_move
  state All_targets_done
    entry:
    DistanceRemainToTarget = single(0);
    doScan = true;
  state Finished
    entry:
    allTargetsDone = true;
    doScan = false;
  (default) -> Standby
  Standby -> Running : [Go == true]
  Running -> All_targets_done : [DistanceRemainToTarget < 7 && TargetIndex >= length(Targets) ]
  Finished -> Running : [~do_one_run]
      | {
      | allTargetsDone = false;
      | TargetIndex = uint8(0);
      | }
  All_targets_done -> Finished : after(3,sec)
  data: BearingRemainToTarget output single size=1; TargetIndex local uint8 size=1 =0; EncoderLeft input int32 size=1; EncoderRight input int32 size=1; DistanceRemainToTarget output single size=1; DistanceCameraTargets input int16; TargetFound local uint8 size=1; BearingCameraTargets input int8; AxleLength parameter single size=1; WheelRadius parameter single size=1; EncRes parameter single size=1; encoder_right_prev_target local int32; ind local uint8; dR local single; dL local single; CurrentDistance local single; CurrentBearing local single; dist_remaining local int16; encoder_left_prev_target local int32; Go input boolean; startPos parameter; Targets input single; prev_target local single; prev_bearing local single; BearingToTarget local single; DistanceToTarget local single; allTargetsDone output boolean; doBeep output boolean; doScan output boolean; pcam parameter; lcam parameter; do_one_run parameter

== stateflow chart SimulationModel/Scoring/Referee/Referee ==
  state Standby
    entry:
    numTargets = size(targetPositions,1);
    targetsFound = false(size(targetPositions,1),1);
    timeLastTargetFound = 0;
    elapsedTime = 0;
    numTargetsFound = 0;
    allowedRunTime = 180;
    startingRadius = 10;
    targetBoundaryRadius = 7;
    statTimeReq = 2.5;
  state Running
    entry: startTiming;
    during:
    elapsedTime = getTiming;
    [nearLocation, currentTarget] = testIfNearLocation(robotPosition, targetPositions, targetBoundaryRadius);
    state NearLocation
      entry: snapshotTime = elapsedTime;
    state Roaming
    Roaming -> NearLocation : [nearLocation == true]
    (default) -> Roaming
    NearLocation -> Roaming [order 2] : [nearLocation == false]
    NearLocation -> (junction 43) [order 1] : [(elapsedTime - snapshotTime) > statTimeReq]
    (junction 44) -> Roaming
    (junction 43) -> (junction 44) : {[targetsFound, timeLastTargetFound] = ...
        | updateTargetsFound(targetsFound, currentTarget, timeLastTargetFound,elapsedTime);
        | numTargetsFound = sum(targetsFound);}
  state Finished
  Finished -> Standby : [StartFlag == false]
  (default) -> Standby
  Standby -> Running : [StartFlag == true &&...
      | distancefrom(robotPosition, startPos) < startingRadius ]
  Running -> Standby [order 2] : [StartFlag == false]
  Running -> Finished [order 1] : [numTargetsFound == numTargets ||...
      |  elapsedTime >= allowedRunTime-sqrt(eps)]
  data: et function_output; tfound_in function_input; currentT function_input; tfound_out function_output; lastTime_in function_input; lastTime_out function_output; time function_input; robotPos function_input; targetPos function_input; proximityVal function_input; nearLoc function_output; currentLoc function_output; pos function_input; x0 function_input; d function_output; startPos parameter; allowedRunTime local; statTimeReq local; startingRadius local; robotPosition input; targetBoundaryRadius local; StartFlag input; targetPositions input; timeLastTargetFound output; nearLocation local; numTargetsFound local; elapsedTime output; numTargets local; currentTarget local; targetsFound output; snapshotTime local; local_t local; sim_time input
  function startTiming:
    | function startTiming
    | global local_t sim_time
    | 
    | if strcmp(coder.target,'rtw')
    |     coder.ceval('tic',int32(2));
    | else
    |     local_t = sim_time;
    | end
  function et = getTiming:
    | function et = getTiming
    | global sim_time local_t
    | 
    | lt = 0;
    | 
    | if strcmp(coder.target,'rtw')
    |     coder.ceval('toc',coder.wref(lt),int32(2));
    | else
    |     lt = sim_time - local_t;
    | end
    | 
    | et = lt;
  function [tfound_out, lastTime_out] = updateTargetsFound(tfound_in, currentT, lastTime_in, time):
    | function [tfound_out, lastTime_out] = updateTargetsFound(tfound_in, currentT, lastTime_in, time)
    | 
    | if any(tfound_in & currentT) %is this an existing target
    |     lastTime_out = lastTime_in;
    | else
    |     lastTime_out = time;
    | end
    | 
    | tfound_out = tfound_in | currentT; %update list of found targets
  function [nearLoc, currentLoc] = testIfNearLocation(robotPos, targetPos, proximityVal):
    | function [nearLoc, currentLoc] = testIfNearLocation(robotPos, targetPos, proximityVal)
    | %#codegen
    | delta = bsxfun(@minus, targetPos, robotPos);
    | dist = sum(delta.^2,2);
    | 
    | currentLoc = dist <= proximityVal^2;
    | nearLoc = any(currentLoc);
  function d = distancefrom(pos,x0):
    | function d = distancefrom(pos,x0)
    | d = sqrt(sum((pos-x0).^2));

== matlab function SimulationModel/Scoring/FigureOutput/call_plotFigure ==
  data: X input; T input; T_found input; t_last input; t input; T_located input; pcam parameter; lcam parameter; robotheta input
function fcn(X, T, T_found, t_last, t, T_located,pcam,lcam,robotheta)
coder.extrinsic('plotFigure');

plotFigure(X, T, T_found, t_last, t, T_located,pcam,lcam,robotheta);

== matlab function SimulationModel/RobotModel/Camera and Image Processing/relative_to_targets ==
  data: robotPos input size=[1 2]; robotTheta input size=1; dist output; bear output; targetsPos input; pcam parameter; lcam parameter
function [dist,bear] = targets(robotPos,robotTheta,targetsPos,pcam,lcam)
%#codegen
%% TARGETS Returns distance and bearing for each target relative to robot
%
% Distances and positions are in cm
% Angles are in degrees
%
% Inputs
%   - hCam: Cam height (from ground)
%   - targetsPos: Position of targets (X,Y)
%   - robotPos: Robot position (X,Y)
%   - robotTheta: Robot angle
%
% Outputs
%   - dist (array nx1 with n=nb targets): Distances for each target, 
%       if a target cannot be seen by the camera associated distance 
%       is equal to -1
%   - bearing (array nx1 with n=nb targets): Angles for each target, 
%       if a target cannot be seen by the camera associated angle is 
%       equal to -1
%

% Get camera field of vision
% [pcam,lcam]=camera(hCam);
% betaCam = 21 ;
% etaCam = 27 ;
% [pcam, lcam] = cameraAnalytic(hCam,90-alphaCam, betaCam, etaCam);

% Convert target position to robot reference
[x,y] = world2robot(robotPos(1),robotPos(2),robotTheta,targetsPos(:,1),targetsPos(:,2));

% Get distance and bearing for each point relative to robot
[distance,bearing] = isincamera(pcam,lcam,x,y);

% sort by descending order and return 6 elements
[distance,idxsort] = sort(distance,'descend');
bearing = bearing(idxsort);
if length(distance)<6
    dist = [distance;zeros(6-length(distance),1)];
    bear = [bearing;zeros(6-length(bearing),1)] ;
else
    dist = distance(1:6);
    bear = bearing(1:6);
end

function [x_new,y_new]=world2robot(x_robot,y_robot,theta_robot,x_world,y_world)
% WORLD2ROBOT Convert coordinates from world to robot
%
% Inputs
%   - x_robot: Robot X position (in world reference)
%   - y_robot: Robot Y position (in world reference)
%   - theta_robot: Robot angle  (in world reference)
%   - x_world: X value(s) to convert (in world reference)
%   - y_world: Y value(s) to convert (in world reference)
%
% Outpus
%   - x_new: Point(s) coordinate (X) in robot reference
%   - y_new: Point(s) coordinate (Y) in robot reference

% Translate coordinates reference
x_dif=x_world-x_robot;
y_dif=y_world-y_robot;

% Rotate coordinates reference
% x_new=x_dif*cosd(theta_robot)-y_dif*sind(theta_robot);
% y_new=x_dif*sind(theta_robot)+y_dif*cosd(theta_robot);
x_new = cosd(theta_robot)*x_dif + sind(theta_robot)*y_dif;
y_new = cosd(theta_robot)*y_dif - sind(theta_robot)*x_dif;
% see http://www.mathematics-online.org/inhalt/aussage/aussage444/

% TODO We have identified that the sign of converted coordinates is the
% opposite of the expected but we don't have an explanation for that
% x_new = -x_new;
% y_new = -y_new;

function [dist,bearing]=isincamera(p,l,x,y)
%% ISINCAMERA Distance and angle from current robot position
%
% Inputs
%   - p (2 elements vector): Minimal and maximal depth for camera (Y axis)
%   - l (2 elements vector): Minimal and maximal width for camera (X axis)
%   - x (vector): X coordinate of point(s)
%   - y (vector): Y coordinate of point(s)
%
% Outputs
%   - dist (vector): Distance of each point from camera (robot), -1 if
%       point cannot be seen by camera.
%   - bearing (vector): Angle of each point from camera (robot), -1 if
%       point cannot be seen by camera.
%

% Calculate coefficients for lines that defines the camera field of vision
% Field vision limits in Y axis are constants (y = p(1) or y = p(2))
c1=polyfit(p(1:2),[-l(1)/2 -l(2)/2],1);
c2=polyfit(p(1:2),[l(1)/2 l(2)/2],1);

% To be visible a point must match all the following criterion
%   - Y >= minimal depth
%   - Y <= maximal depth
%   - X >= - (width for current Y) / 2
%   - X <=   (width for current Y) / 2
%

%isvisible = y>=p(1) & y<=p(2) & (x>=polyval(c1,y) & x<=polyval(c2,y));
isvisible = x>=p(1) & x<=p(2) & (y>=polyval(c1,x) & y<=polyval(c2,x));

% Calculate distance and bearing for all points
dist = sqrt(x.^2 + y.^2);
% bearing = atan2d(y,x);
bearing = atan2d(x,-y)-90;

% Replace values by -1 for points that are not visible
dist(~isvisible) = 0;
bearing(~isvisible) = 0;

== matlab function SimulationModel/RobotModel/Camera and Image Processing/dist_bearing2locatedTargets ==
  data: robotPos input; dist input; locatedTargets output; bearing input; robotTheta input
function locatedTargets = fcn(robotPos, dist, bearing, robotTheta)
%#codegen

loc = dist > 0;

locatedTargetsX = zeros(size(dist));
locatedTargetsY = locatedTargetsX;

targetTheta = robotTheta + bearing(loc);

locatedTargetsX(loc) = robotPos(1) + dist(loc) .* cosd(targetTheta);
locatedTargetsY(loc) = robotPos(2) + dist(loc) .* sind(targetTheta);

locatedTargets = [locatedTargetsX, locatedTargetsY];
